simulink model "PMSM_model"  (R2016b)
settings: Solver=VariableStepAuto  StartTime=0.0  StopTime=10.0  RelTol=1e-3  EnableMultiTasking=on
values from neighbouring files (symbols this model uses):
  Ampmax = 400*sqrt(2)/sqrt(3)*3/2    [parameters.m]
  J = 0.0334    [parameters.m]
  ki = 100    [parameters.m]
  kp = 1000    [parameters.m]
  L_s = 0.0173    [parameters.m]
  p = 6    [parameters.m]
  Psi_R = 3*T_rated/sqrt(2)/p/I_rated    [parameters.m]
  R_s = 5.05    [parameters.m]
  T23 = [2/3 0; -1/3 1/sqrt(3); -1/3 -1/sqrt(3)]    [parameters.m]
  T32 = [1 -1/2 -1/2; 0 sqrt(3)/2 -sqrt(3)/2 ]    [parameters.m]
undefined symbols (not defined in the file or in its folder): j
libraries: simulink x2
settings Model: Creator=martin  LastModifiedBy=martin
settings DataIOCC: LimitDataPoints=on
settings OptimizationCC: LifeSpan=inf
settings DebuggingCC: AllowSymbolicDim=off  SFUnexpectedBacktrackingDiag=warning  SFNoUnconditionalDefaultTransitionDiag=warning  SFExecutionAtInitializationDiag=none
settings ModelReferenceCC: PropagateSignalLabelsOutOfModel=off
settings GRTTargetCC: TargetLangStandard=C89/C90 (ANSI)
settings ConfigComp: CovMetricSettings=dw  CovHtmlReporting=on  CovSaveCumulativeToWorkspaceVar=on  CovSaveSingleToWorkspaceVar=on  CovExternalEMLEnable=off

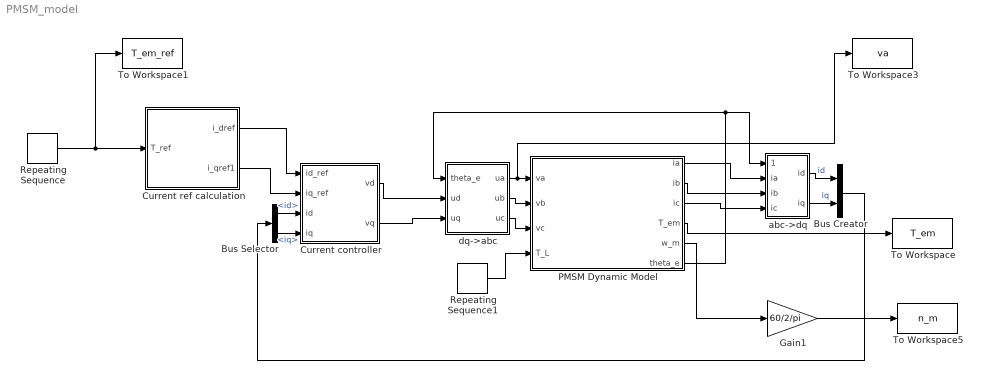
== system PMSM_model ==
  Bus Creator : BusCreator  Inputs=2
  Bus Selector : BusSelector  OutputSignals=id,iq
  Current controller : Subsystem
  Current ref calculation : Subsystem
  Gain1 : Gain  Gain=60/2/pi
  PMSM Dynamic Model : Subsystem
  Repeating Sequence : simulink/Sources/Repeating Sequence  rep_seq_t=[0 1 2 3 4 5 6 7 8 9 10 11]  rep_seq_y=[0 1 1 1 0 -1 -1 -1 0 1 1 1]*0.1 + 0.3*[0 1 1 1 1 1 1 1 1 1 1 1]
  Repeating Sequence1 : simulink/Sources/Repeating Sequence  rep_seq_t=[0 1 2 3 4 5 6 7 8 10]  rep_seq_y=0.3*[0 1 1 1 1 1 1 1 1 1]
  To Workspace : ToWorkspace  VariableName=T_em  SaveFormat=Timeseries  SampleTime=-1
  To Workspace1 : ToWorkspace  VariableName=T_em_ref  SaveFormat=Timeseries  SampleTime=-1
  To Workspace3 : ToWorkspace  VariableName=va  SaveFormat=Timeseries  SampleTime=-1
  To Workspace5 : ToWorkspace  VariableName=n_m  SaveFormat=Timeseries  SampleTime=-1
  abc->dq : Subsystem
  dq->abc : Subsystem
  wires:
  PMSM Dynamic Model/1(ia) -> abc->dq/2(ia)
  PMSM Dynamic Model/2(ib) -> abc->dq/3(ib)
  PMSM Dynamic Model/3(ic) -> abc->dq/4(ic)
  dq->abc/1(ua) -> To Workspace3/1, PMSM Dynamic Model/1(va)
  dq->abc/2(ub) -> PMSM Dynamic Model/2(vb)
  dq->abc/3(uc) -> PMSM Dynamic Model/3(vc)
  Repeating Sequence1/1 -> PMSM Dynamic Model/4(T_L)
  abc->dq/1(id) -> Bus Creator/1  "id"
  abc->dq/2(iq) -> Bus Creator/2  "iq"
  Bus Creator/1 -> Bus Selector/1
  Current ref calculation/1(i_dref) -> Current controller/1(id_ref)
  Current ref calculation/2(i_qref1) -> Current controller/2(iq_ref)
  Bus Selector/1 -> Current controller/3(id)  "<id>"
  Bus Selector/2 -> Current controller/4(iq)  "<iq>"
  Current controller/1(vd) -> dq->abc/2(ud)
  Current controller/2(vq) -> dq->abc/3(uq)
  PMSM Dynamic Model/5(w_m) -> Gain1/1
  PMSM Dynamic Model/4(T_em) -> To Workspace/1
  Repeating Sequence/1 -> To Workspace1/1, Current ref calculation/1(T_ref)
  Gain1/1 -> To Workspace5/1
  PMSM Dynamic Model/6(theta_e) -> dq->abc/1("theta_e "), abc->dq/1(theta_e)

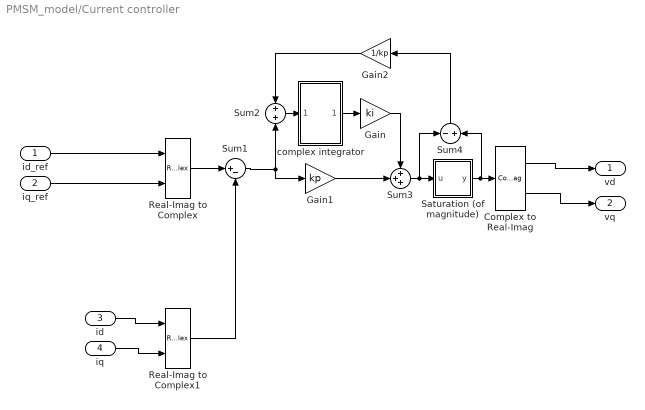
== system PMSM_model/Current controller ==
  id_ref : Inport
  iq_ref : Inport  Port=2
  id : Inport  Port=3
  iq : Inport  Port=4
  Complex to Real-Imag : ComplexToRealImag
  Gain : Gain  Gain=ki
  Gain1 : Gain  Gain=kp
  Gain2 : Gain  Gain=1/kp
  Real-Imag to Complex : RealImagToComplex
  Real-Imag to Complex1 : RealImagToComplex
  Saturation (of magnitude) : Subsystem
      mask Display: disp('sat');
  Sum1 : Sum  Inputs=|+-  SaturateOnIntegerOverflow=on  InputSameDT=on  OutDataTypeStr=Inherit: Same as first input
  Sum2 : Sum  Inputs=+|+  SaturateOnIntegerOverflow=on  InputSameDT=on  OutDataTypeStr=Inherit: Same as first input
  Sum3 : Sum  Inputs=+++  SaturateOnIntegerOverflow=on  InputSameDT=on  OutDataTypeStr=Inherit: Same as first input
  Sum4 : Sum  Inputs=-+  SaturateOnIntegerOverflow=on  InputSameDT=on  OutDataTypeStr=Inherit: Same as first input
  complex integrator : Subsystem
  vd : Outport
  vq : Outport  Port=2
  wires:
  complex integrator/1(Out1) -> Gain/1
  id/1 -> Real-Imag to Complex1/1
  Sum2/1 -> complex integrator/1(In1)
  Sum3/1 -> Sum4/1, Saturation (of magnitude)/1(u)
  Complex to Real-Imag/1 -> vd/1
  id_ref/1 -> Real-Imag to Complex/1
  Real-Imag to Complex/1 -> Sum1/1
  Saturation (of magnitude)/1(y) -> Sum4/2, Complex to Real-Imag/1
  iq_ref/1 -> Real-Imag to Complex/2
  Gain2/1 -> Sum2/1
  Sum1/1 -> Sum2/2, Gain1/1
  iq/1 -> Real-Imag to Complex1/2
  Complex to Real-Imag/2 -> vq/1
  Gain/1 -> Sum3/1
  Gain1/1 -> Sum3/2
  Real-Imag to Complex1/1 -> Sum1/2
  Sum4/1 -> Gain2/1

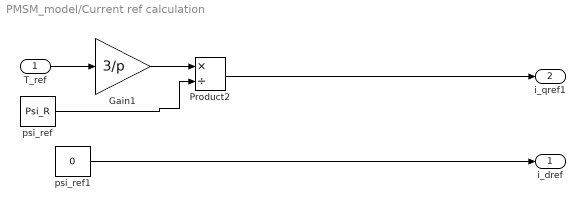
== system PMSM_model/Current ref calculation ==
  T_ref : Inport
  Gain1 : Gain  Gain=3/p
  Product2 : Product  Inputs=*/  RndMeth=Zero
  psi_ref : Constant  Value=Psi_R
  psi_ref1 : Constant  Value=0
  i_dref : Outport
  i_qref1 : Outport  Port=2
  wires:
  psi_ref/1 -> Product2/2
  Product2/1 -> i_qref1/1
  T_ref/1 -> Gain1/1
  Gain1/1 -> Product2/1
  psi_ref1/1 -> i_dref/1

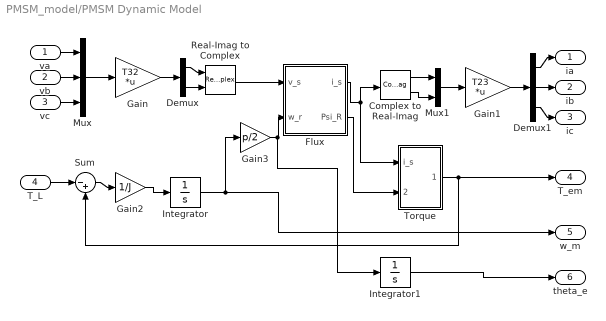
== system PMSM_model/PMSM Dynamic Model ==
  va : Inport
  vb : Inport  Port=2
  vc : Inport  Port=3
  T_L : Inport  Port=4
  Complex to Real-Imag : ComplexToRealImag
  Demux : Demux  Outputs=2
  Demux1 : Demux  Outputs=3
  Flux : Subsystem
  Gain : Gain  Gain=T32  Multiplication=Matrix(K*u)
  Gain1 : Gain  Gain=T23  Multiplication=Matrix(K*u)
  Gain2 : Gain  Gain=1/J
  Gain3 : Gain  Gain=p/2
  Integrator : Integrator
  Integrator1 : Integrator
  Mux : Mux  Inputs=3
  Mux1 : Mux  Inputs=2
  Real-Imag to Complex : RealImagToComplex
  Sum : Sum  Inputs=|-+
  Torque : Subsystem
  ia : Outport
  ib : Outport  Port=2
  ic : Outport  Port=3
  T_em : Outport  Port=4
  w_m : Outport  Port=5
  theta_e : Outport  Port=6
  wires:
  va/1 -> Mux/1
  Mux1/1 -> Gain1/1
  Mux/1 -> Gain/1
  Demux1/3 -> ic/1
  vb/1 -> Mux/2
  Complex to Real-Imag/1 -> Mux1/1
  vc/1 -> Mux/3
  Demux/2 -> Real-Imag to Complex/2
  Complex to Real-Imag/2 -> Mux1/2
  Gain/1 -> Demux/1
  Gain3/1 -> Integrator1/1, Flux/2(w_r)
  Demux1/1 -> ia/1
  Demux1/2 -> ib/1
  Real-Imag to Complex/1 -> Flux/1(v_s)
  Flux/1(i_s) -> Complex to Real-Imag/1, Torque/1(i_s)
  Gain1/1 -> Demux1/1
  Demux/1 -> Real-Imag to Complex/1
  Flux/2(Psi_R) -> Torque/2(Psi_R)
  Integrator/1 -> w_m/1, Gain3/1
  Gain2/1 -> Integrator/1
  Sum/1 -> Gain2/1
  Torque/1(T_em) -> T_em/1, Sum/2
  T_L/1 -> Sum/1
  Integrator1/1 -> theta_e/1

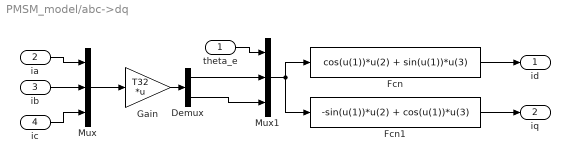
== system PMSM_model/abc->dq ==
  theta_e : Inport
  ia : Inport  Port=2
  ib : Inport  Port=3
  ic : Inport  Port=4
  Demux : Demux  Outputs=2
  Fcn : Fcn  Expr=cos(u(1))*u(2) + sin(u(1))*u(3)
  Fcn1 : Fcn  Expr=-sin(u(1))*u(2) + cos(u(1))*u(3)
  Gain : Gain  Gain=T32  Multiplication=Matrix(K*u)
  Mux : Mux  Inputs=3
  Mux1 : Mux  Inputs=3
  id : Outport
  iq : Outport  Port=2
  wires:
  ic/1 -> Mux/3
  ib/1 -> Mux/2
  Gain/1 -> Demux/1
  ia/1 -> Mux/1
  Mux/1 -> Gain/1
  Demux/1 -> Mux1/2
  Demux/2 -> Mux1/3
  Mux1/1 -> Fcn1/1, Fcn/1
  Fcn/1 -> id/1
  Fcn1/1 -> iq/1
  theta_e/1 -> Mux1/1

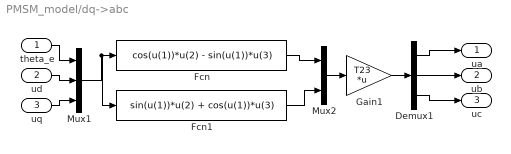
== system PMSM_model/dq->abc ==
  "theta_e " : Inport
  ud : Inport  Port=2
  uq : Inport  Port=3
  Demux1 : Demux  Outputs=3
  Fcn : Fcn  Expr=cos(u(1))*u(2) - sin(u(1))*u(3)
  Fcn1 : Fcn  Expr=sin(u(1))*u(2) + cos(u(1))*u(3)
  Gain1 : Gain  Gain=T23  Multiplication=Matrix(K*u)
  Mux1 : Mux  Inputs=3
  Mux2 : Mux  Inputs=2
  ua : Outport
  ub : Outport  Port=2
  uc : Outport  Port=3
  wires:
  Demux1/3 -> uc/1
  Gain1/1 -> Demux1/1
  Demux1/2 -> ub/1
  Demux1/1 -> ua/1
  Mux2/1 -> Gain1/1
  Mux1/1 -> Fcn1/1, Fcn/1
  Fcn/1 -> Mux2/1
  Fcn1/1 -> Mux2/2
  "theta_e "/1 -> Mux1/1
  ud/1 -> Mux1/2
  uq/1 -> Mux1/3

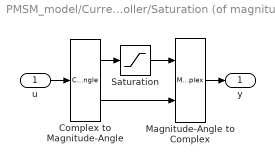
== system PMSM_model/Current controller/Saturation (of magnitude) ==
  u : Inport
  Complex to Magnitude-Angle : ComplexToMagnitudeAngle
  Magnitude-Angle to Complex : MagnitudeAngleToComplex
  Saturation : Saturate  UpperLimit=Ampmax  LowerLimit=0  LinearizeAsGain=off
  y : Outport
  wires:
  u/1 -> Complex to Magnitude-Angle/1
  Magnitude-Angle to Complex/1 -> y/1
  Saturation/1 -> Magnitude-Angle to Complex/1
  Complex to Magnitude-Angle/2 -> Magnitude-Angle to Complex/2
  Complex to Magnitude-Angle/1 -> Saturation/1

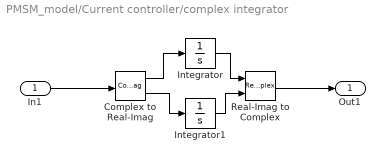
== system PMSM_model/Current controller/complex integrator ==
  In1 : Inport
  Complex to Real-Imag : ComplexToRealImag
  Integrator : Integrator
  Integrator1 : Integrator
  Real-Imag to Complex : RealImagToComplex
  Out1 : Outport
  wires:
  Integrator1/1 -> Real-Imag to Complex/2
  Complex to Real-Imag/1 -> Integrator/1
  Real-Imag to Complex/1 -> Out1/1
  Integrator/1 -> Real-Imag to Complex/1
  Complex to Real-Imag/2 -> Integrator1/1
  In1/1 -> Complex to Real-Imag/1

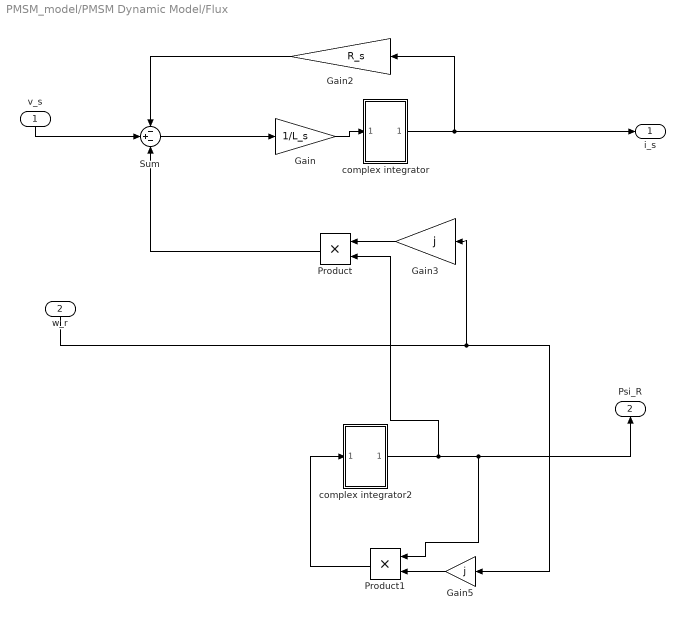
== system PMSM_model/PMSM Dynamic Model/Flux ==
  v_s : Inport
  w_r : Inport  Port=2
  Gain : Gain  Gain=1/L_s
  Gain2 : Gain  Gain=R_s
  Gain3 : Gain  Gain=j
  Gain5 : Gain  Gain=j
  Product : Product
  Product1 : Product
  Sum : Sum  Inputs=-+-
  complex integrator : Subsystem
  complex integrator2 : Subsystem
  i_s : Outport
  Psi_R : Outport  Port=2
  wires:
  complex integrator/1(Out1) -> i_s/1, Gain2/1
  Gain3/1 -> Product/1
  Gain/1 -> complex integrator/1(In1)
  Sum/1 -> Gain/1
  Product/1 -> Sum/3
  Gain2/1 -> Sum/1
  v_s/1 -> Sum/2
  complex integrator2/1(Out1) -> Product/2, Product1/1, Psi_R/1
  w_r/1 -> Gain5/1, Gain3/1
  Gain5/1 -> Product1/2
  Product1/1 -> complex integrator2/1(In1)

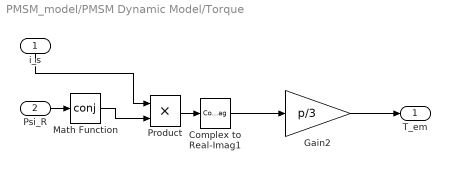
== system PMSM_model/PMSM Dynamic Model/Torque ==
  i_s : Inport
  Psi_R : Inport  Port=2
  Complex to Real-Imag1 : ComplexToRealImag  Output=Imag
  Gain2 : Gain  Gain=p/3
  Math Function : Math  Operator=conj  SaturateOnIntegerOverflow=on
  Product : Product
  T_em : Outport
  wires:
  Product/1 -> Complex to Real-Imag1/1
  Math Function/1 -> Product/2
  Psi_R/1 -> Math Function/1
  i_s/1 -> Product/1
  Gain2/1 -> T_em/1
  Complex to Real-Imag1/1 -> Gain2/1

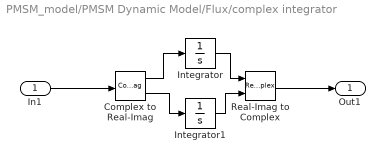
== system PMSM_model/PMSM Dynamic Model/Flux/complex integrator ==
  In1 : Inport
  Complex to Real-Imag : ComplexToRealImag
  Integrator : Integrator
  Integrator1 : Integrator
  Real-Imag to Complex : RealImagToComplex
  Out1 : Outport
  wires:
  Integrator1/1 -> Real-Imag to Complex/2
  Complex to Real-Imag/1 -> Integrator/1
  Real-Imag to Complex/1 -> Out1/1
  Integrator/1 -> Real-Imag to Complex/1
  Complex to Real-Imag/2 -> Integrator1/1
  In1/1 -> Complex to Real-Imag/1

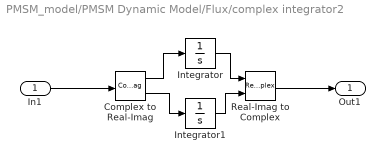
== system PMSM_model/PMSM Dynamic Model/Flux/complex integrator2 ==
  In1 : Inport
  Complex to Real-Imag : ComplexToRealImag
  Integrator : Integrator  InitialCondition=Psi_R
  Integrator1 : Integrator
  Real-Imag to Complex : RealImagToComplex
  Out1 : Outport
  wires:
  In1/1 -> Complex to Real-Imag/1
  Complex to Real-Imag/2 -> Integrator1/1
  Integrator/1 -> Real-Imag to Complex/1
  Real-Imag to Complex/1 -> Out1/1
  Complex to Real-Imag/1 -> Integrator/1
  Integrator1/1 -> Real-Imag to Complex/2
